simulink subsystem "trial"  (R2023a)
settings: Solver=VariableStepAuto  StartTime=0.0  StopTime=10.0  RelTol=1e-3
undefined symbols (not defined in the file or in its folder): Btrigger_boost, DAapply_nudges, DAdesired_pose, DAff_body_force, DAsolver_weights, Djoy_R_X, Dreverse_throttle, Dthrottle, Iangular_mode, Ilinear_mode
libraries: ros2lib x76
settings Model: Creator=john  LastModifiedBy=john

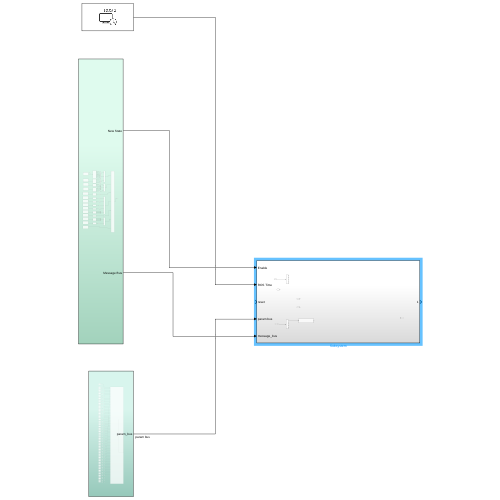
[thumbnail: Simulink's stored preview of the top-level diagram]
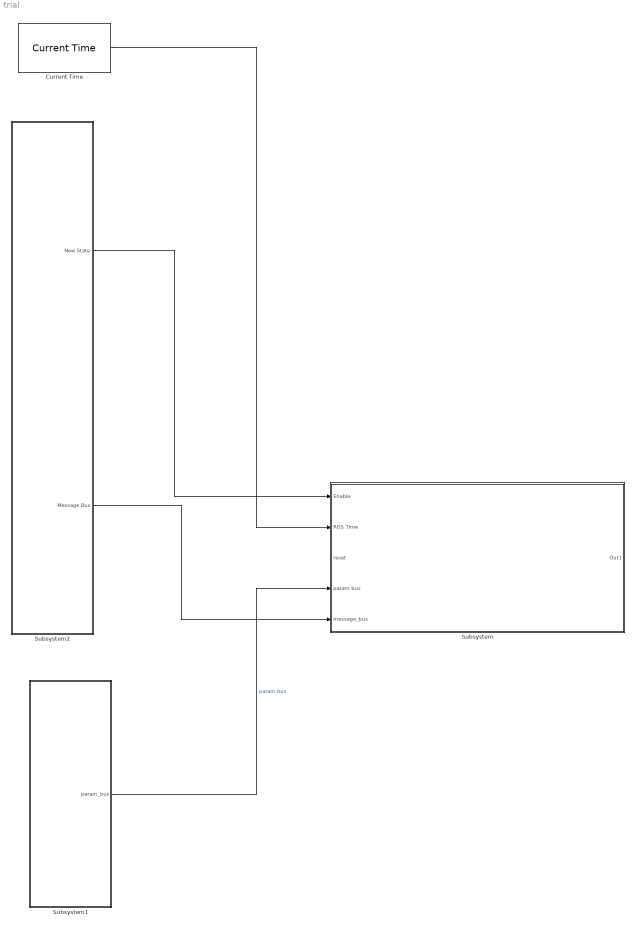
== system trial ==
  Current Time : ros2lib/Current Time  OutputFormat=double  SampleTime=-1  ModelName=complete_controller
  Subsystem : Subsystem
  Subsystem1 : Subsystem
  Subsystem2 : Subsystem
  wires:
  Subsystem2/2(Message Bus) -> Subsystem/5(message_bus)
  Subsystem1/1(param_bus) -> Subsystem/4(param bus)  "param bus"
  Current Time/1 -> Subsystem/2(ROS Time)
  Subsystem2/1(New State) -> Subsystem/1(Enable)

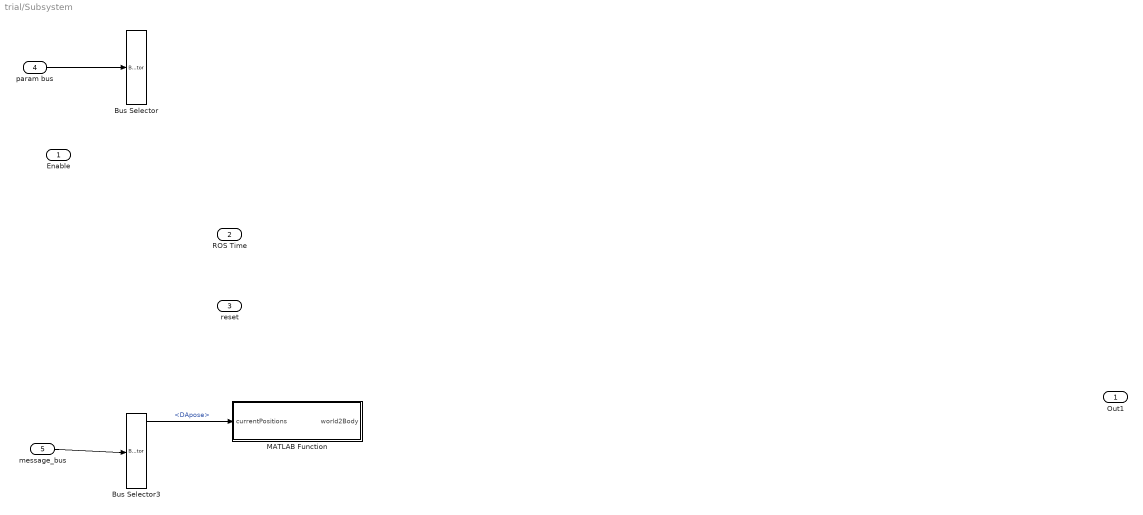
== system trial/Subsystem ==
  Enable : Inport
  ROS Time : Inport  Port=2
  reset : Inport  Port=3
  param bus : Inport  Port=4
  message_bus : Inport  Port=5
  Bus Selector : BusSelector  OutputSignals=DAmax_control,DAp_gains,DAd_gains,DAi_gains,Dreset_threshold
  Bus Selector3 : BusSelector  OutputSignals=current_state.DApose,current_state.DAtwist,desired_pose.DAdesired_pose,Bmotion_enabled
  MATLAB Function : MATLAB Function  TreatAsAtomicUnit=on
  Out1 : Outport
  wires:
  param bus/1 -> Bus Selector/1
  message_bus/1 -> Bus Selector3/1
  Bus Selector3/1 -> MATLAB Function/1(currentPositions)  "<DApose>"

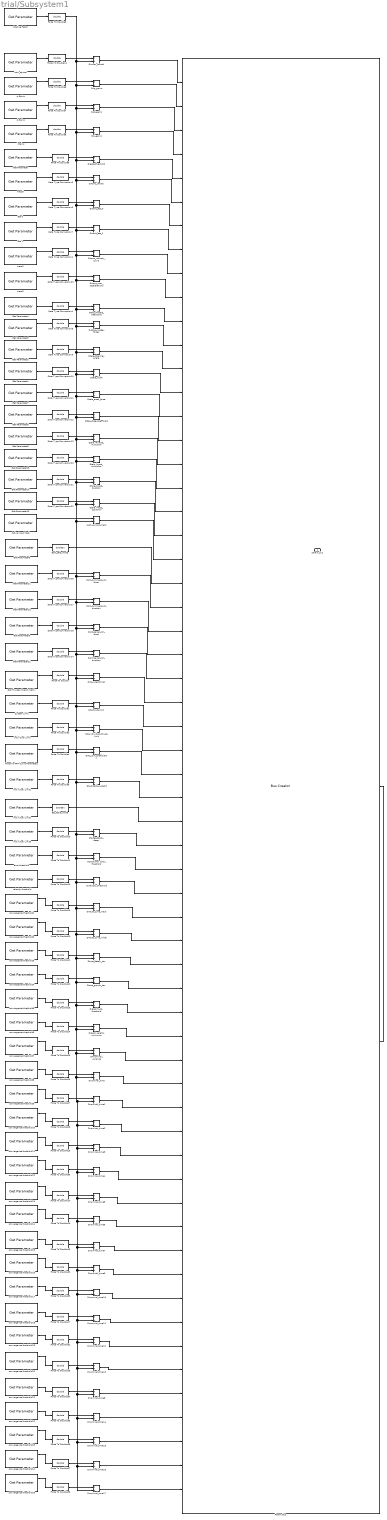
== system trial/Subsystem1 ==
  Active Input Mask : ros2lib/Get Parameter  ParameterName=controller__active_force_mask  ParameterType=int64[]  ParameterMaxArrayLength=6  ParameterInitialValue=[0,0,0,0,0,0]  SampleTime=-1  ModelName=complete_controller  BlockId=ParamGet_complete_controller_223
  Bsnt_safe_mode : DataTypeConversion  OutDataTypeStr=boolean  SaturateOnIntegerOverflow=off  RndMeth=Floor
  Bts_table_mode : DataTypeConversion  OutDataTypeStr=boolean  SaturateOnIntegerOverflow=off  RndMeth=Floor
  DAauto_tune_initial : Product  Inputs=*/
  DAauto_tune_mask : Product  Inputs=*/
  DAd_gains : Product  Inputs=*/
  DAi_gains : Product  Inputs=*/
  DAmax_control : Product  Inputs=*/
  DAnominal_variance : Product  Inputs=*/
  DAp_gains : Product  Inputs=*/
  DAsmc_eta_0 : Product  Inputs=*/
  DAsmc_eta_1 : Product  Inputs=*/
  DAsmc_lamda : Product  Inputs=*/
  DAsmc_max_accelerations : Product  Inputs=*/
  DAsmc_velocity_curve : Product  Inputs=*/
  DAtele_nudge_forces : Product  Inputs=*/
  DAts_rpm_coefficients : Product  Inputs=*/
  DAts_wrenchmat : Product  Inputs=*/
  Data Type Conversion{1,4..14,16..18,20..23} (19 alike) : DataTypeConversion  OutDataTypeStr=double  SaturateOnIntegerOverflow=off  RndMeth=Floor
  Dnominal_time{,1..17} (18 alike) : Product  Inputs=*/
  Dpositional_error_threshold : Product  Inputs=*/
  Dreset_threshold : Product  Inputs=*/
  Dreset_trust_threshold : Product  Inputs=*/
  Dreset_weight_minimum : Product  Inputs=*/
  Dsnt_barrel_roll_duration : Product  Inputs=*/
  Dsnt_barrel_roll_force : Product  Inputs=*/
  Dsnt_summersault_duration : Product  Inputs=*/
  Dsnt_summersault_force : Product  Inputs=*/
  Dtele_accel_force : Product  Inputs=*/
  Dtele_boost_cooldown : Product  Inputs=*/
  Dtele_boost_duration : Product  Inputs=*/
  Dtele_boost_multiplier : Product  Inputs=*/
  Dtele_drag_coefficient : Product  Inputs=*/
  Dtele_reverse_multiplier : Product  Inputs=*/
  Dtele_steering_angle : Product  Inputs=*/
  Dtele_throttle_deadzone : Product  Inputs=*/
  Dtele_width : Product  Inputs=*/
  Dtrust_decay_tau : Product  Inputs=*/
  Dtrust_growth_tau : Product  Inputs=*/
  Dts_disable_weight : Product  Inputs=*/
  Dts_feedback_decay : Product  Inputs=*/
  Dts_individual_thrust_limit : Product  Inputs=*/
  Dts_thrust_limit : Product  Inputs=*/
  Dvelocity_threshold : Product  Inputs=*/
  Eta 0 : ros2lib/Get Parameter  ParameterName=controller__SMC__SMC_params__eta_order_0  ParameterType=int64[]  ParameterMaxArrayLength=6  ParameterInitialValue=0.0  SampleTime=-1  ModelName=complete_controller  BlockId=ParamGet_complete_controller_274
      settings: LibrarySourceBlock=roslib/ROS 2/Get Parameter
  Eta 1 : ros2lib/Get Parameter  ParameterName=controller__SMC__SMC_params__eta_order_1  ParameterType=int64[]  ParameterMaxArrayLength=6  ParameterInitialValue=0.0  SampleTime=-1  ModelName=complete_controller  BlockId=ParamGet_complete_controller_275
      settings: LibrarySourceBlock=roslib/ROS 2/Get Parameter
  Force To Double{,1..38} (39 alike) : DataTypeConversion  OutDataTypeStr=double  SaturateOnIntegerOverflow=off  RndMeth=Floor
  Force To RPM Curve Parameters : ros2lib/Get Parameter  ParameterName=thruster_solver__force_to_rpm_coefficents  ParameterType=int64[]  ParameterMaxArrayLength=8  ParameterInitialValue=[0,0,0,0,0,0,0,0]  SampleTime=-1  ModelName=complete_controller  BlockId=ParamGet_complete_controller_190
      settings: LibrarySourceBlock=roslib/ROS 2/Get Parameter
  Get Parameter : ros2lib/Get Parameter  ParameterName=controller__pid__reset_threshold  ParameterType=int64  ParameterMaxArrayLength=16  ParameterInitialValue=100000  SampleTime=-1  ModelName=complete_controller  BlockId=ParamGet_complete_controller_251
      settings: LibrarySourceBlock=roslib/ROS 2/Get Parameter
  Get Parameter1 : ros2lib/Get Parameter  ParameterName=controller__teleop__width  ParameterType=int64  ParameterMaxArrayLength=16  ParameterInitialValue=900000  SampleTime=-1  ModelName=complete_controller  BlockId=ParamGet_complete_controller_382
  Get Parameter10 : ros2lib/Get Parameter  ParameterName=controller__stunt__summersault_duration  ParameterType=int64  ParameterMaxArrayLength=16  ParameterInitialValue=5000000.0  SampleTime=-1  ModelName=complete_controller  BlockId=ParamGet_complete_controller_425
  Get Parameter11 : ros2lib/Get Parameter  ParameterName=controller__stunt__summersault_force  ParameterType=int64  ParameterMaxArrayLength=16  ParameterInitialValue=20000000  SampleTime=-1  ModelName=complete_controller  BlockId=ParamGet_complete_controller_426
  Get Parameter12 : ros2lib/Get Parameter  ParameterName=controller__stunt__barrel_roll_duration  ParameterType=int64  ParameterMaxArrayLength=16  ParameterInitialValue=4000000.0  SampleTime=-1  ModelName=complete_controller  BlockId=ParamGet_complete_controller_427
  Get Parameter13 : ros2lib/Get Parameter  ParameterName=controller__teleop__boost__cooldown  ParameterType=int64  ParameterMaxArrayLength=16  ParameterInitialValue=10000000  SampleTime=-1  ModelName=complete_controller  BlockId=ParamGet_complete_controller_460
  Get Parameter14 : ros2lib/Get Parameter  ParameterName=controller__teleop__boost__duration  ParameterType=int64  ParameterMaxArrayLength=16  ParameterInitialValue=5000000  SampleTime=-1  ModelName=complete_controller  BlockId=ParamGet_complete_controller_461
  Get Parameter15 : ros2lib/Get Parameter  ParameterName=controller__teleop__boost__multiplier  ParameterType=int64  ParameterMaxArrayLength=16  ParameterInitialValue=1500000  SampleTime=-1  ModelName=complete_controller  BlockId=ParamGet_complete_controller_462
  Get Parameter2 : ros2lib/Get Parameter  ParameterName=controller__teleop__max_steering_angle  ParameterType=int64  ParameterMaxArrayLength=16  ParameterInitialValue=45000000  SampleTime=-1  ModelName=complete_controller  BlockId=ParamGet_complete_controller_383
  Get Parameter3 : ros2lib/Get Parameter  ParameterName=controller__teleop__nudge_forces  ParameterType=int64[]  ParameterMaxArrayLength=6  ParameterInitialValue=[20000000, 20000000, 2000000, 200000, 200000, 2000000]  SampleTime=-1  ModelName=complete_controller  BlockId=ParamGet_complete_controller_384
  Get Parameter4 : ros2lib/Get Parameter  ParameterName=controller__teleop__throttle_deadzone  ParameterType=int64  ParameterMaxArrayLength=16  ParameterInitialValue=50000  SampleTime=-1  ModelName=complete_controller  BlockId=ParamGet_complete_controller_385
  Get Parameter5 : ros2lib/Get Parameter  ParameterName=controller__teleop__reverse_force_multiplier  ParameterType=int64  ParameterMaxArrayLength=16  ParameterInitialValue=400000  SampleTime=-1  ModelName=complete_controller  BlockId=ParamGet_complete_controller_386
  Get Parameter6 : ros2lib/Get Parameter  ParameterName=controller__teleop__drag_coefficient  ParameterType=int64  ParameterMaxArrayLength=16  ParameterInitialValue=420000000  SampleTime=-1  ModelName=complete_controller  BlockId=ParamGet_complete_controller_387
  Get Parameter7 : ros2lib/Get Parameter  ParameterName=controller__teleop__accel_force  ParameterType=int64  ParameterMaxArrayLength=16  ParameterInitialValue=20000000  SampleTime=-1  ModelName=complete_controller  BlockId=ParamGet_complete_controller_388
  Get Parameter8 : ros2lib/Get Parameter  ParameterName=controller__stunt__safe_mode  ParameterType=boolean  ParameterMaxArrayLength=16  ParameterInitialValue=0  SampleTime=-1  ModelName=complete_controller  BlockId=ParamGet_complete_controller_423
  Get Parameter9 : ros2lib/Get Parameter  ParameterName=controller__stunt__barrel_roll_force  ParameterType=int64  ParameterMaxArrayLength=16  ParameterInitialValue=25000000.0  SampleTime=-1  ModelName=complete_controller  BlockId=ParamGet_complete_controller_424
  Get Thruster Wrench Matrix : ros2lib/Get Parameter  ParameterName=talos_wrenchmat  ParameterType=int64[]  ParameterMaxArrayLength=48  ParameterInitialValue=0.0  SampleTime=-1  ModelName=complete_controller  BlockId=ParamGet_complete_controller_191
      settings: LibrarySourceBlock=roslib/ROS 2/Get Parameter
  Iactive_input_mask : Product  Inputs=*/
  Individual Limit : ros2lib/Get Parameter  ParameterName=thruster_solver__individual_thrust_limit  ParameterType=int64  ParameterMaxArrayLength=16  ParameterInitialValue=5.0  SampleTime=-1  ModelName=complete_controller  BlockId=ParamGet_complete_controller_192
      settings: LibrarySourceBlock=roslib/ROS 2/Get Parameter
  Individual Limit1 : ros2lib/Get Parameter  ParameterName=thruster_solver__disable_weight  ParameterType=int64  ParameterMaxArrayLength=16  ParameterInitialValue=10000000  SampleTime=-1  ModelName=complete_controller  BlockId=ParamGet_complete_controller_193
      settings: LibrarySourceBlock=roslib/ROS 2/Get Parameter
  Individual Limit2 : ros2lib/Get Parameter  ParameterName=thruster_solver_table_mode  ParameterType=boolean  ParameterMaxArrayLength=16  ParameterInitialValue=false  SampleTime=-1  ModelName=complete_controller  BlockId=ParamGet_complete_controller_194
      settings: LibrarySourceBlock=roslib/ROS 2/Get Parameter
  Individual Limit3 : ros2lib/Get Parameter  ParameterName=thruster_solver__feedback_decay  ParameterType=int64  ParameterMaxArrayLength=16  ParameterInitialValue=1250000  SampleTime=-1  ModelName=complete_controller  BlockId=ParamGet_complete_controller_486
      settings: LibrarySourceBlock=roslib/ROS 2/Get Parameter
  Param Bus : BusCreator  Inputs=60
  Scaling Factor : ros2lib/Get Parameter  ParameterName=controller__SMC__SMC_params__scaling_factor  ParameterType=int64  ParameterMaxArrayLength=16  ParameterInitialValue=1000000  SampleTime=-1  ModelName=complete_controller  BlockId=ParamGet_complete_controller_219
      settings: LibrarySourceBlock=roslib/ROS 2/Get Parameter
  System Limit : ros2lib/Get Parameter  ParameterName=thruster_solver__system_thrust_limit  ParameterType=int64  ParameterMaxArrayLength=16  ParameterInitialValue=10  SampleTime=-1  ModelName=complete_controller  BlockId=ParamGet_complete_controller_221
      settings: LibrarySourceBlock=roslib/ROS 2/Get Parameter
  convergence threshold1 : ros2lib/Get Parameter  ParameterName=controller__feed_forward__auto_tune__auto_tune_mask  ParameterType=int64[]  ParameterMaxArrayLength=6  ParameterInitialValue=[0;0;0;0;0;0]  SampleTime=-1  ModelName=complete_controller  BlockId=ParamGet_complete_controller_725
      settings: LibrarySourceBlock=roslib/ROS 2/Get Parameter
  convergence threshold10 : ros2lib/Get Parameter  ParameterName=controller__feed_forward__auto_tune__trust_threshold  ParameterType=int64[]  ParameterMaxArrayLength=6  ParameterInitialValue=[970000, 970000, 970000, 970000, 970000, 970000]  SampleTime=-1  ModelName=complete_controller  BlockId=ParamGet_complete_controller_814
      settings: LibrarySourceBlock=roslib/ROS 2/Get Parameter
  convergence threshold11 : ros2lib/Get Parameter  ParameterName=controller__feed_forward__auto_tune__variation_threshold  ParameterType=int64[]  ParameterMaxArrayLength=6  ParameterInitialValue=[1000000, 1000000, 1000000, 1000000, 1000000, 1000000]  SampleTime=-1  ModelName=complete_controller  BlockId=ParamGet_complete_controller_817
      settings: LibrarySourceBlock=roslib/ROS 2/Get Parameter
  convergence threshold12 : ros2lib/Get Parameter  ParameterName=controller__feed_forward__auto_tune__axis_weights  ParameterType=int64[]  ParameterMaxArrayLength=6  ParameterInitialValue=[1000000, 1000000, 1000000, 1000000, 1000000, 1000000]  SampleTime=-1  ModelName=complete_controller  BlockId=ParamGet_complete_controller_820
      settings: LibrarySourceBlock=roslib/ROS 2/Get Parameter
  convergence threshold13 : ros2lib/Get Parameter  ParameterName=controller__feed_forward__auto_tune__variation_der_threshold  ParameterType=int64[]  ParameterMaxArrayLength=6  ParameterInitialValue=[1000000, 1000000, 1000000, 1000000, 1000000, 1000000]  SampleTime=-1  ModelName=complete_controller  BlockId=ParamGet_complete_controller_830
      settings: LibrarySourceBlock=roslib/ROS 2/Get Parameter
  convergence threshold14 : ros2lib/Get Parameter  ParameterName=inertia  ParameterType=int64[]  ParameterMaxArrayLength=3  ParameterInitialValue=[700000,1590000,1650000]  SampleTime=-1  ModelName=complete_controller  BlockId=ParamGet_complete_controller_911
      settings: LibrarySourceBlock=roslib/ROS 2/Get Parameter
  convergence threshold15 : ros2lib/Get Parameter  ParameterName=mass  ParameterType=int64  ParameterMaxArrayLength=6  ParameterInitialValue=32000000  SampleTime=-1  ModelName=complete_controller  BlockId=ParamGet_complete_controller_912
      settings: LibrarySourceBlock=roslib/ROS 2/Get Parameter
  convergence threshold16 : ros2lib/Get Parameter  ParameterName=controller__drag_compensator__apply_mask  ParameterType=int64[]  ParameterMaxArrayLength=36  ParameterInitialValue=zeros(36,1)  SampleTime=-1  ModelName=complete_controller  BlockId=ParamGet_complete_controller_971
      settings: LibrarySourceBlock=roslib/ROS 2/Get Parameter
  convergence threshold17 : ros2lib/Get Parameter  ParameterName=controller__drag_compensator__minimum_samples  ParameterType=int64  ParameterMaxArrayLength=6  ParameterInitialValue=60000000  SampleTime=-1  ModelName=complete_controller  BlockId=ParamGet_complete_controller_972
      settings: LibrarySourceBlock=roslib/ROS 2/Get Parameter
  convergence threshold18 : ros2lib/Get Parameter  ParameterName=controller__drag_compensator__minimum_absolute_velocity  ParameterType=int64  ParameterMaxArrayLength=6  ParameterInitialValue=200000  SampleTime=-1  ModelName=complete_controller  BlockId=ParamGet_complete_controller_973
      settings: LibrarySourceBlock=roslib/ROS 2/Get Parameter
  convergence threshold19 : ros2lib/Get Parameter  ParameterName=controller__drag_compensator__minimum_absolute_positional_error  ParameterType=int64  ParameterMaxArrayLength=3  ParameterInitialValue=200000  SampleTime=-1  ModelName=complete_controller  BlockId=ParamGet_complete_controller_974
      settings: LibrarySourceBlock=roslib/ROS 2/Get Parameter
  convergence threshold2 : ros2lib/Get Parameter  ParameterName=auto_ff__auto_ff  ParameterType=int64[]  ParameterMaxArrayLength=6  ParameterInitialValue=[0;0;0;0;0;0]  SampleTime=-1  ModelName=complete_controller  BlockId=ParamGet_complete_controller_730
      settings: LibrarySourceBlock=roslib/ROS 2/Get Parameter
  convergence threshold20 : ros2lib/Get Parameter  ParameterName=controller__drag_compensator__minimum_average_sampled_velocity  ParameterType=int64[]  ParameterMaxArrayLength=6  ParameterInitialValue=[100000,100000,100000,100000,100000,100000]  SampleTime=-1  ModelName=complete_controller  BlockId=ParamGet_complete_controller_975
      settings: LibrarySourceBlock=roslib/ROS 2/Get Parameter
  convergence threshold21 : ros2lib/Get Parameter  ParameterName=controller__drag_compensator__minimum_R2_coeffiecent  ParameterType=int64  ParameterMaxArrayLength=6  ParameterInitialValue=700000  SampleTime=-1  ModelName=complete_controller  BlockId=ParamGet_complete_controller_978
      settings: LibrarySourceBlock=roslib/ROS 2/Get Parameter
  convergence threshold22 : ros2lib/Get Parameter  ParameterName=controller__drag_compensator__learning_rate  ParameterType=int64  ParameterMaxArrayLength=6  ParameterInitialValue=200000  SampleTime=-1  ModelName=complete_controller  BlockId=ParamGet_complete_controller_981
      settings: LibrarySourceBlock=roslib/ROS 2/Get Parameter
  convergence threshold23 : ros2lib/Get Parameter  ParameterName=controller__drag_compensator__initial_compensation__forward  ParameterType=int64[]  ParameterMaxArrayLength=36  ParameterInitialValue=zeros(36,1)  SampleTime=-1  ModelName=complete_controller  BlockId=ParamGet_complete_controller_1006
      settings: LibrarySourceBlock=roslib/ROS 2/Get Parameter
  convergence threshold24 : ros2lib/Get Parameter  ParameterName=controller__autoff__initial_ff  ParameterType=int64[]  ParameterMaxArrayLength=6  ParameterInitialValue=[0,0,0,0,0,0,0]  SampleTime=-1  ModelName=complete_controller  BlockId=ParamGet_complete_controller_1009
      settings: LibrarySourceBlock=roslib/ROS 2/Get Parameter
  convergence threshold25 : ros2lib/Get Parameter  ParameterName=controller__drag_compensator__initial_compensation__reverse  ParameterType=int64[]  ParameterMaxArrayLength=36  ParameterInitialValue=zeros(36,1)  SampleTime=-1  ModelName=complete_controller  BlockId=ParamGet_complete_controller_1030
      settings: LibrarySourceBlock=roslib/ROS 2/Get Parameter
  convergence threshold3 : ros2lib/Get Parameter  ParameterName=controller__controller_scale__trust_decay_tau  ParameterType=int64  ParameterMaxArrayLength=6  ParameterInitialValue=1000000  SampleTime=-1  ModelName=complete_controller  BlockId=ParamGet_complete_controller_760
      settings: LibrarySourceBlock=roslib/ROS 2/Get Parameter
  convergence threshold4 : ros2lib/Get Parameter  ParameterName=controller__controller_scale__trust_growth_tau  ParameterType=int64  ParameterMaxArrayLength=6  ParameterInitialValue=1000000  SampleTime=-1  ModelName=complete_controller  BlockId=ParamGet_complete_controller_763
      settings: LibrarySourceBlock=roslib/ROS 2/Get Parameter
  convergence threshold5 : ros2lib/Get Parameter  ParameterName=controller__controller_scale__reset_trust_threshold  ParameterType=int64  ParameterMaxArrayLength=200000  ParameterInitialValue=200000  SampleTime=-1  ModelName=complete_controller  BlockId=ParamGet_complete_controller_766
      settings: LibrarySourceBlock=roslib/ROS 2/Get Parameter
  convergence threshold6 : ros2lib/Get Parameter  ParameterName=controller__controller_scale__reset_weight_minimum  ParameterType=int64  ParameterMaxArrayLength=6  ParameterInitialValue=3000000  SampleTime=-1  ModelName=complete_controller  BlockId=ParamGet_complete_controller_769
      settings: LibrarySourceBlock=roslib/ROS 2/Get Parameter
  convergence threshold7 : ros2lib/Get Parameter  ParameterName=controller__controller_scale__nominal_variance  ParameterType=int64[]  ParameterMaxArrayLength=6  ParameterInitialValue=[0;0;0;0;0;0]  SampleTime=-1  ModelName=complete_controller  BlockId=ParamGet_complete_controller_772
      settings: LibrarySourceBlock=roslib/ROS 2/Get Parameter
  convergence threshold8 : ros2lib/Get Parameter  ParameterName=controller__controller_scale__nominal_time  ParameterType=int64  ParameterMaxArrayLength=6  ParameterInitialValue=3000000  SampleTime=-1  ModelName=complete_controller  BlockId=ParamGet_complete_controller_775
      settings: LibrarySourceBlock=roslib/ROS 2/Get Parameter
  convergence threshold9 : ros2lib/Get Parameter  ParameterName=controller__feed_forward__auto_tune__decay_factor  ParameterType=int64[]  ParameterMaxArrayLength=6  ParameterInitialValue=[200000, 200000, 200000, 200000, 200000, 200000]  SampleTime=-1  ModelName=complete_controller  BlockId=ParamGet_complete_controller_805
      settings: LibrarySourceBlock=roslib/ROS 2/Get Parameter
  d Gains : ros2lib/Get Parameter  ParameterName=controller__PID__d_gains  ParameterType=int64[]  ParameterMaxArrayLength=6  ParameterInitialValue=[0,0,0,0,0,0]  SampleTime=-1  ModelName=complete_controller  BlockId=ParamGet_complete_controller_260
      settings: LibrarySourceBlock=roslib/ROS 2/Get Parameter
  error threshold : ros2lib/Get Parameter  ParameterName=controller__feed_forward__auto_tune__positional_error_threshold  ParameterType=int64  ParameterMaxArrayLength=16  ParameterInitialValue=100000  SampleTime=-1  ModelName=complete_controller  BlockId=ParamGet_complete_controller_702
      settings: LibrarySourceBlock=roslib/ROS 2/Get Parameter
  i Gains : ros2lib/Get Parameter  ParameterName=controller__PID__i_gains  ParameterType=int64[]  ParameterMaxArrayLength=6  ParameterInitialValue=[0,0,0,0,0,0]  SampleTime=-1  ModelName=complete_controller  BlockId=ParamGet_complete_controller_261
      settings: LibrarySourceBlock=roslib/ROS 2/Get Parameter
  mass1 : ros2lib/Get Parameter  ParameterName=controller__SMC__SMC_params__velocity_curve_params  ParameterType=int64[]  ParameterMaxArrayLength=12  ParameterInitialValue=[0,0,0,0,0,0,0,0,0,0,0,0]  SampleTime=-1  ModelName=complete_controller  BlockId=ParamGet_complete_controller_276
      settings: LibrarySourceBlock=roslib/ROS 2/Get Parameter
  mass2 : ros2lib/Get Parameter  ParameterName=controller__SMC__max_target_accelerations  ParameterType=int64[]  ParameterMaxArrayLength=6  ParameterInitialValue=[10000,10000,10000,10000,10000,10000]  SampleTime=-1  ModelName=complete_controller  BlockId=ParamGet_complete_controller_467
      settings: LibrarySourceBlock=roslib/ROS 2/Get Parameter
  mass5 : ros2lib/Get Parameter  ParameterName=controller__SMC__SMC_params__lambda  ParameterType=int64[]  ParameterMaxArrayLength=6  ParameterInitialValue=0.0  SampleTime=-1  ModelName=complete_controller  BlockId=ParamGet_complete_controller_278
      settings: LibrarySourceBlock=roslib/ROS 2/Get Parameter
  max_control : ros2lib/Get Parameter  ParameterName=controller__PID__max_control_thresholds  ParameterType=int64[]  ParameterMaxArrayLength=6  ParameterInitialValue=[0,0,0,0,0,0]  SampleTime=-1  ModelName=complete_controller  BlockId=ParamGet_complete_controller_262
      settings: LibrarySourceBlock=roslib/ROS 2/Get Parameter
  p Gains : ros2lib/Get Parameter  ParameterName=controller__PID__p_gains  ParameterType=int64[]  ParameterMaxArrayLength=6  ParameterInitialValue=[0,0,0,0,0,0]  SampleTime=-1  ModelName=complete_controller  BlockId=ParamGet_complete_controller_263
      settings: LibrarySourceBlock=roslib/ROS 2/Get Parameter
  velocity threshold : ros2lib/Get Parameter  ParameterName=controller__feed_forward__auto_tune__velocity_threshold  ParameterType=int64  ParameterMaxArrayLength=16  ParameterInitialValue=100000  SampleTime=-1  ModelName=complete_controller  BlockId=ParamGet_complete_controller_703
      settings: LibrarySourceBlock=roslib/ROS 2/Get Parameter
  param_bus : Outport
  wires:
  Data Type Conversion10/1 -> Dtele_width/1
  Get Parameter4/1 -> Data Type Conversion4/1
  Data Type Conversion22/1 -> Dtele_boost_cooldown/1
  Data Type Conversion20/1 -> Dtele_boost_multiplier/1
  Data Type Conversion11/1 -> Dtele_accel_force/1
  Data Type Conversion23/1 -> DAsmc_max_accelerations/1
  Get Parameter11/1 -> Data Type Conversion16/1
  Get Parameter5/1 -> Data Type Conversion13/1
  Force To RPM Curve Parameters/1 -> Force To Double4/1
  Data Type Conversion13/1 -> Dtele_reverse_multiplier/1
  Get Parameter7/1 -> Data Type Conversion11/1
  Get Parameter1/1 -> Data Type Conversion10/1
  Data Type Conversion21/1 -> Dtele_boost_duration/1
  Get Parameter12/1 -> Data Type Conversion14/1
  Data Type Conversion16/1 -> Dsnt_summersault_force/1
  Scaling Factor/1 -> Force To Double3/1
  Get Parameter6/1 -> Data Type Conversion12/1
  Eta 0/1 -> Data Type Conversion6/1
  Data Type Conversion7/1 -> DAsmc_eta_1/1
  Individual Limit/1 -> Force To Double2/1
  Data Type Conversion8/1 -> DAtele_nudge_forces/1
  Force To Double6/1 -> DAp_gains/1
  p Gains/1 -> Force To Double6/1
  Force To Double5/1 -> Dts_disable_weight/1
  Get Thruster Wrench Matrix/1 -> Force To Double/1
  Get Parameter10/1 -> Data Type Conversion17/1
  Data Type Conversion18/1 -> Dsnt_barrel_roll_force/1
  max_control/1 -> Force To Double11/1
  mass2/1 -> Data Type Conversion23/1
  Get Parameter13/1 -> Data Type Conversion22/1
  Data Type Conversion14/1 -> Dsnt_barrel_roll_duration/1
  Force To Double8/1 -> DAi_gains/1
  Active Input Mask/1 -> Iactive_input_mask/1
  Eta 1/1 -> Data Type Conversion7/1
  Force To Double7/1 -> DAd_gains/1
  Data Type Conversion12/1 -> Dtele_drag_coefficient/1
  d Gains/1 -> Force To Double7/1
  Force To Double4/1 -> DAts_rpm_coefficients/1
  Get Parameter9/1 -> Data Type Conversion18/1
  Get Parameter8/1 -> Bsnt_safe_mode/1
  Individual Limit1/1 -> Force To Double5/1
  Data Type Conversion5/1 -> DAsmc_lamda/1
  mass1/1 -> Data Type Conversion1/1
  Get Parameter/1 -> Force To Double9/1
  Data Type Conversion9/1 -> Dtele_steering_angle/1
  Individual Limit3/1 -> Force To Double10/1
  Get Parameter14/1 -> Data Type Conversion21/1
  mass5/1 -> Data Type Conversion5/1
  System Limit/1 -> Force To Double1/1
  Get Parameter3/1 -> Data Type Conversion8/1
  i Gains/1 -> Force To Double8/1
  Force To Double11/1 -> DAmax_control/1
  Data Type Conversion1/1 -> DAsmc_velocity_curve/1
  Get Parameter15/1 -> Data Type Conversion20/1
  Force To Double1/1 -> Dts_thrust_limit/1
  Data Type Conversion4/1 -> Dtele_throttle_deadzone/1
  Get Parameter2/1 -> Data Type Conversion9/1
  Force To Double9/1 -> Dreset_threshold/1
  Force To Double2/1 -> Dts_individual_thrust_limit/1
  Force To Double10/1 -> Dts_feedback_decay/1
  Data Type Conversion17/1 -> Dsnt_summersault_duration/1
  Data Type Conversion6/1 -> DAsmc_eta_0/1
  Force To Double/1 -> DAts_wrenchmat/1
  Individual Limit2/1 -> Bts_table_mode/1
  Dts_feedback_decay/1 -> Param Bus/33  "Dts_feedback_decay"
  Bts_table_mode/1 -> Param Bus/32  "Bts_table_mode"
  Dts_disable_weight/1 -> Param Bus/31  "Dts_disable_weight"
  DAts_rpm_coefficients/1 -> Param Bus/30  "DAts_rpm_coefficients"
  Dts_individual_thrust_limit/1 -> Param Bus/29  "Dts_individual_thrust_limit"
  Dts_thrust_limit/1 -> Param Bus/28  "Dts_thrust_limit"
  DAts_wrenchmat/1 -> Param Bus/27  "DAts_wrenchmat"
  Dsnt_barrel_roll_duration/1 -> Param Bus/26  "Dsnt_barrel_roll_duration"
  Bsnt_safe_mode/1 -> Param Bus/22  "Bsnt_safe_mode"
  Dsnt_barrel_roll_force/1 -> Param Bus/25  "Dsnt_barrel_roll_force"
  Dsnt_summersault_duration/1 -> Param Bus/24  "Dsnt_summersault_duration"
  Dsnt_summersault_force/1 -> Param Bus/23  "Dsnt_summersault_force"
  Iactive_input_mask/1 -> Param Bus/21  "Iactive_input_mask"
  Dtele_boost_cooldown/1 -> Param Bus/20  "Dtele_boost_cooldown"
  Dtele_boost_duration/1 -> Param Bus/19  "Dtele_boost_duration"
  Dtele_boost_multiplier/1 -> Param Bus/18  "Dtele_boost_multiplier"
  Dtele_reverse_multiplier/1 -> Param Bus/17  "Dtele_reverse_multiplier"
  Dtele_drag_coefficient/1 -> Param Bus/16  "Dtele_drag_coefficient"
  Dtele_accel_force/1 -> Param Bus/15  "Dtele_accel_force"
  Dtele_width/1 -> Param Bus/14  "Dtele_width"
  Dtele_steering_angle/1 -> Param Bus/13  "Dtele_steering_angle"
  DAtele_nudge_forces/1 -> Param Bus/12  "DAtele_nudge_forces"
  Dtele_throttle_deadzone/1 -> Param Bus/11  "Dtele_throttle_deadzone"
  DAsmc_max_accelerations/1 -> Param Bus/10  "DAsmc_max_accelerations"
  DAsmc_velocity_curve/1 -> Param Bus/9  "DAsmc_velocity_curve"
  DAsmc_eta_1/1 -> Param Bus/8  "DAsmc_eta_1"
  DAsmc_eta_0/1 -> Param Bus/7  "DAsmc_eta_0"
  DAsmc_lamda/1 -> Param Bus/6  "DAsmc_lamda"
  Dreset_threshold/1 -> Param Bus/5  "Dreset_threshold"
  DAi_gains/1 -> Param Bus/4  "DAi_gains"
  DAd_gains/1 -> Param Bus/3  "DAd_gains"
  DAp_gains/1 -> Param Bus/2  "DAp_gains"
  DAmax_control/1 -> Param Bus/1  "DAmax_control"
  Param Bus/1 -> param_bus/1
  error threshold/1 -> Force To Double12/1
  velocity threshold/1 -> Force To Double13/1
  Dpositional_error_threshold/1 -> Param Bus/34  "Dpositional_error_threshold"
  Dvelocity_threshold/1 -> Param Bus/35  "Dvelocity_threshold"
  convergence threshold1/1 -> Force To Double19/1
  DAauto_tune_mask/1 -> Param Bus/36  "DAauto_tune_mask"
  Force To Double13/1 -> Dvelocity_threshold/1
  Force To Double12/1 -> Dpositional_error_threshold/1
  Force To Double19/1 -> DAauto_tune_mask/1
  convergence threshold2/1 -> Force To Double20/1
  DAauto_tune_initial/1 -> Param Bus/37  "DAauto_tune_initial"
  Force To Double20/1 -> DAauto_tune_initial/1
  convergence threshold3/1 -> Force To Double21/1
  Dtrust_decay_tau/1 -> Param Bus/38  "Dtrust_decay_tau"
  Force To Double21/1 -> Dtrust_decay_tau/1
  convergence threshold4/1 -> Force To Double22/1
  Dtrust_growth_tau/1 -> Param Bus/39  "Dtrust_growth_tau"
  Force To Double22/1 -> Dtrust_growth_tau/1
  convergence threshold5/1 -> Force To Double23/1
  Dreset_trust_threshold/1 -> Param Bus/40  "Dreset_trust_threshold"
  Force To Double23/1 -> Dreset_trust_threshold/1
  convergence threshold6/1 -> Force To Double24/1
  Dreset_weight_minimum/1 -> Param Bus/41  "Dreset_weight_minimum"
  Force To Double24/1 -> Dreset_weight_minimum/1
  convergence threshold7/1 -> Force To Double25/1
  DAnominal_variance/1 -> Param Bus/42  "DAnominal_variance"
  Force To Double25/1 -> DAnominal_variance/1
  convergence threshold8/1 -> Force To Double26/1
  Dnominal_time/1 -> Param Bus/43  "Dnominal_time"
  Force To Double26/1 -> Dnominal_time/1
  convergence threshold9/1 -> Force To Double27/1
  Force To Double27/1 -> Dnominal_time1/1
  convergence threshold10/1 -> Force To Double28/1
  Force To Double28/1 -> Dnominal_time2/1
  convergence threshold11/1 -> Force To Double29/1
  Force To Double29/1 -> Dnominal_time3/1
  convergence threshold12/1 -> Force To Double30/1
  Force To Double30/1 -> Dnominal_time4/1
  Dnominal_time1/1 -> Param Bus/44  "DAautoff_body_force_decay_percentage"
  Dnominal_time2/1 -> Param Bus/45  "DAautoff_measurement_trust_threshold"
  Dnominal_time3/1 -> Param Bus/46  "DAautoff_standard_variation_threshold"
  Dnominal_time4/1 -> Param Bus/47  "DAautoff_active_force_weights"
  convergence threshold13/1 -> Force To Double14/1
  Force To Double14/1 -> Dnominal_time5/1
  Dnominal_time5/1 -> Param Bus/48  "DAautoff_variation_derivative_threshold"
  Force To Double16/1 -> Dnominal_time6/1
  Dnominal_time6/1 -> Param Bus/49  "DAinterias"
  convergence threshold15/1 -> Force To Double15/1
  Dnominal_time7/1 -> Param Bus/50  "Dmass"
  Force To Double15/1 -> Dnominal_time7/1
  convergence threshold14/1 -> Force To Double16/1
  Dnominal_time13/1 -> Param Bus/55  "DAminimum_drag_update_velocity"
  convergence threshold20/1 -> Force To Double18/1
  Dnominal_time10/1 -> Param Bus/52  "Iminimum_drag_samples"
  Force To Double31/1 -> Dnominal_time12/1
  Dnominal_time11/1 -> Param Bus/53  "Dminimum_drag_sampling_velocity"
  convergence threshold19/1 -> Force To Double31/1
  convergence threshold18/1 -> Force To Double17/1
  Force To Double33/1 -> Dnominal_time10/1
  Dnominal_time12/1 -> Param Bus/54  "Dminimum_drag_positional_error"
  Dnominal_time9/1 -> Param Bus/51  "IAdrag_apply_mask"
  Force To Double17/1 -> Dnominal_time11/1
  convergence threshold17/1 -> Force To Double33/1
  Force To Double32/1 -> Dnominal_time9/1
  convergence threshold16/1 -> Force To Double32/1
  Force To Double18/1 -> Dnominal_time13/1
  convergence threshold21/1 -> Force To Double34/1
  Force To Double34/1 -> Dnominal_time8/1
  Dnominal_time8/1 -> Param Bus/56  "Ddrag_minimum_correspondence_coeffiecent"
  convergence threshold22/1 -> Force To Double35/1
  Dnominal_time14/1 -> Param Bus/57  "Ddrag_learning_rate"
  Force To Double35/1 -> Dnominal_time14/1
  convergence threshold23/1 -> Force To Double36/1
  Dnominal_time15/1 -> Param Bus/58  "DAdrag_init_compensation_forward"
  Force To Double36/1 -> Dnominal_time15/1
  Dnominal_time16/1 -> Param Bus/59  "DAautoff_init_compensation"
  Force To Double37/1 -> Dnominal_time16/1
  convergence threshold24/1 -> Force To Double37/1
  Force To Double3/1 -> Dtele_throttle_deadzone/2, DAtele_nudge_forces/2, Dtele_steering_angle/2, Dtele_width/2, Dtele_accel_force/2, Dtele_drag_coefficient/2, Dtele_boost_multiplier/2, Dtele_boost_duration/2, Dtele_boost_cooldown/2, Dsnt_summersault_force/2, Dsnt_summersault_duration/2, Dsnt_barrel_roll_duration/2, DAts_wrenchmat/2, Dts_thrust_limit/2, Dts_individual_thrust_limit/2, DAts_rpm_coefficients/2, Dvelocity_threshold/2, Dtrust_decay_tau/2, Dtrust_growth_tau/2, Dreset_trust_threshold/2, Dreset_weight_minimum/2, DAnominal_variance/2, Dnominal_time17/2, Dnominal_time16/2, Dnominal_time15/2, Dnominal_time14/2, Dnominal_time8/2, Dnominal_time13/2, Dnominal_time12/2, Dnominal_time11/2, Dnominal_time10/2, Dnominal_time9/2, Dnominal_time7/2, Dnominal_time6/2, Dnominal_time5/2, Dnominal_time4/2, Dnominal_time3/2, Dnominal_time2/2, Dnominal_time1/2, Dnominal_time/2, DAauto_tune_initial/2, DAauto_tune_mask/2, Dpositional_error_threshold/2, Dts_feedback_decay/2, Dts_disable_weight/2, Dsnt_barrel_roll_force/2, Iactive_input_mask/2, Dtele_reverse_multiplier/2, DAsmc_max_accelerations/2, DAsmc_velocity_curve/2, DAsmc_eta_1/2, DAsmc_eta_0/2, DAsmc_lamda/2, Dreset_threshold/2, DAi_gains/2, DAd_gains/2, DAp_gains/2, DAmax_control/2
  Force To Double38/1 -> Dnominal_time17/1
  convergence threshold25/1 -> Force To Double38/1
  Dnominal_time17/1 -> Param Bus/60  "DAdrag_init_compensation_reverse"

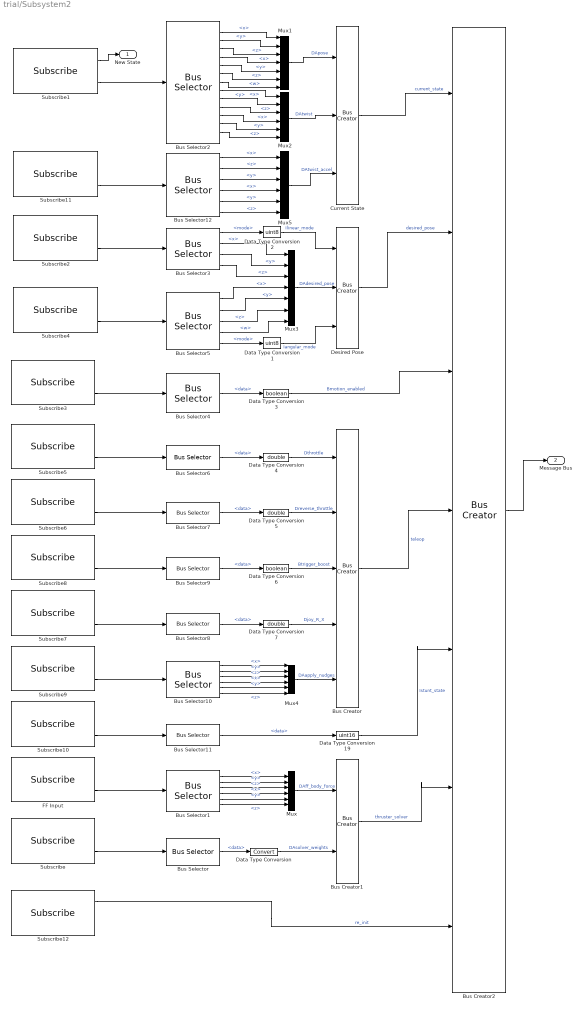
== system trial/Subsystem2 ==
  Bus Creator : BusCreator  Inputs=Dthrottle,Dreverse_throttle,Btrigger_boost,Djoy_R_X,DAapply_nudges
  Bus Creator1 : BusCreator  Inputs=DAff_body_force,DAsolver_weights
  Bus Creator2 : BusCreator  Inputs=7
  Bus Selector{,4,6..9,11} (7 alike) : BusSelector  OutputSignals=data
  Bus Selector1 : BusSelector  OutputSignals=linear.x,linear.y,linear.z,angular.x,angular.y,angular.z
  Bus Selector10 : BusSelector  OutputSignals=linear.x,linear.y,linear.z,angular.x,angular.y,angular.z
  Bus Selector12 : BusSelector  OutputSignals=accel.accel.linear.x,accel.accel.linear.z,accel.accel.linear.y,accel.accel.angular.x,accel.accel.angular.y,accel.accel.angular.z
  Bus Selector2 : BusSelector  OutputSignals=pose.pose.position.x,pose.pose.position.y,pose.pose.position.z,pose.pose.orientation.x,pose.pose.orientation.y,pose.pose.orientation.z,pose.pose.orientation.w,twist.twist.linear.x,twist.twist.linear.y,twist.twist.linear.z,twist.twist.angular.x,twist.twist.angular.y,twist.twist.angular.z
  Bus Selector3 : BusSelector  OutputSignals=mode,setpoint_vect.x,setpoint_vect.y,setpoint_vect.z
  Bus Selector5 : BusSelector  OutputSignals=setpoint_quat.x,setpoint_quat.y,setpoint_quat.z,setpoint_quat.w,mode
  Current State : BusCreator  Inputs=3
  Data Type Conversion : DataTypeConversion  SaturateOnIntegerOverflow=off  RndMeth=Floor
  Data Type Conversion1 : DataTypeConversion  OutDataTypeStr=uint8  SaturateOnIntegerOverflow=off  RndMeth=Floor
  Data Type Conversion19 : DataTypeConversion  OutDataTypeStr=uint16  SaturateOnIntegerOverflow=off  RndMeth=Floor
  Data Type Conversion2 : DataTypeConversion  OutDataTypeStr=uint8  SaturateOnIntegerOverflow=off  RndMeth=Floor
  Data Type Conversion3 : DataTypeConversion  OutDataTypeStr=boolean  SaturateOnIntegerOverflow=off  RndMeth=Floor
  Data Type Conversion4 : DataTypeConversion  OutDataTypeStr=double  SaturateOnIntegerOverflow=off  RndMeth=Floor
  Data Type Conversion5 : DataTypeConversion  OutDataTypeStr=double  SaturateOnIntegerOverflow=off  RndMeth=Floor
  Data Type Conversion6 : DataTypeConversion  OutDataTypeStr=boolean  SaturateOnIntegerOverflow=off  RndMeth=Floor
  Data Type Conversion7 : DataTypeConversion  OutDataTypeStr=double  SaturateOnIntegerOverflow=off  RndMeth=Floor
  Desired Pose : BusCreator  Inputs=Ilinear_mode,DAdesired_pose,Iangular_mode
  FF Input : ros2lib/Subscribe  topicSource=Specify your own  topic=/talos/controller/FF_body_force  messageType=geometry_msgs/Twist  sampleTime=-1  QOSHistory=Keep last  QOSDepth=1  QOSReliability=Reliable  QOSDurability=Volatile
      settings: LibrarySourceBlock=roslib/ROS 2/Subscribe
  Mux{,2,4..5} (4 alike) : Mux  Inputs=6
  Mux1 : Mux  Inputs=7
  Mux3 : Mux  Inputs=7
  Subscribe : ros2lib/Subscribe  topicSource=Specify your own  topic=/talos/controller/solver_weights  messageType=std_msgs/Int32MultiArray  sampleTime=-1  QOSHistory=Keep last  QOSDepth=1  QOSReliability=Reliable  QOSDurability=Volatile
      settings: LibrarySourceBlock=roslib/ROS 2/Subscribe
  Subscribe1 : ros2lib/Subscribe  topicSource=Specify your own  topic=/talos/odometry/filtered  messageType=nav_msgs/Odometry  sampleTime=-1  QOSHistory=Keep last  QOSDepth=1  QOSReliability=Reliable  QOSDurability=Volatile
      settings: LibrarySourceBlock=roslib/ROS 2/Subscribe
  Subscribe10 : ros2lib/Subscribe  topicSource=Specify your own  topic=/talos/controller/stunt_state  messageType=std_msgs/UInt16  sampleTime=-1  QOSHistory=Keep last  QOSDepth=1  QOSReliability=Reliable  QOSDurability=Volatile
  Subscribe11 : ros2lib/Subscribe  topicSource=Specify your own  topic=/talos/accel/filtered  messageType=geometry_msgs/AccelWithCovarianceStamped  sampleTime=-1  QOSHistory=Keep last  QOSDepth=1  QOSReliability=Reliable  QOSDurability=Volatile
      settings: LibrarySourceBlock=roslib/ROS 2/Subscribe
  Subscribe12 : ros2lib/Subscribe  topicSource=Specify your own  topic=/talos/controller/re_init_accumulators  messageType=std_msgs/Empty  sampleTime=-1  QOSHistory=Keep last  QOSDepth=1  QOSReliability=Reliable  QOSDurability=Volatile
      settings: LibrarySourceBlock=roslib/ROS 2/Subscribe
  Subscribe2 : ros2lib/Subscribe  topicSource=Specify your own  topic=/talos/controller/linear  messageType=riptide_msgs2/ControllerCommand  sampleTime=-1  QOSHistory=Keep last  QOSDepth=1  QOSReliability=Reliable  QOSDurability=Volatile
      settings: LibrarySourceBlock=roslib/ROS 2/Subscribe
  Subscribe3 : ros2lib/Subscribe  topicSource=Specify your own  topic=/talos/controller/motion_enabled  messageType=std_msgs/Bool  sampleTime=-1  QOSHistory=Keep last  QOSDepth=1  QOSReliability=Reliable  QOSDurability=Volatile
      settings: LibrarySourceBlock=roslib/ROS 2/Subscribe
  Subscribe4 : ros2lib/Subscribe  topicSource=Specify your own  topic=/talos/controller/angular  messageType=riptide_msgs2/ControllerCommand  sampleTime=-1  QOSHistory=Keep last  QOSDepth=1  QOSReliability=Reliable  QOSDurability=Volatile
      settings: LibrarySourceBlock=roslib/ROS 2/Subscribe
  Subscribe5 : ros2lib/Subscribe  topicSource=Specify your own  topic=/talos/teleop/throttle  messageType=std_msgs/Float32  sampleTime=-1  QOSHistory=Keep last  QOSDepth=5  QOSReliability=Best effort  QOSDurability=Volatile
  Subscribe6 : ros2lib/Subscribe  topicSource=Specify your own  topic=/talos/teleop/reverse  messageType=std_msgs/Float32  sampleTime=-1  QOSHistory=Keep last  QOSDepth=5  QOSReliability=Best effort  QOSDurability=Volatile
  Subscribe7 : ros2lib/Subscribe  topicSource=Specify your own  topic=/talos/teleop/joy_R_X  messageType=std_msgs/Float32  sampleTime=-1  QOSHistory=Keep last  QOSDepth=5  QOSReliability=Best effort  QOSDurability=Volatile
  Subscribe8 : ros2lib/Subscribe  topicSource=Specify your own  topic=/talos/teleop/trigger_boost  messageType=std_msgs/Bool  sampleTime=-1  QOSHistory=Keep last  QOSDepth=1  QOSReliability=Reliable  QOSDurability=Volatile
  Subscribe9 : ros2lib/Subscribe  topicSource=Specify your own  topic=/talos/teleop/apply_nudges  messageType=geometry_msgs/Twist  sampleTime=-1  QOSHistory=Keep last  QOSDepth=5  QOSReliability=Best effort  QOSDurability=Volatile
  New State : Outport
  Message Bus : Outport  Port=2
  wires:
  Bus Selector1/1 -> Mux/1  "<x>"
  Bus Selector2/4 -> Mux1/4  "<x>"
  Mux/1 -> Bus Creator1/1  "DAff_body_force"
  Bus Selector2/12 -> Mux2/5  "<y>"
  Bus Selector11/1 -> Data Type Conversion19/1  "<data>"
  Subscribe4/2 -> Bus Selector5/1
  Bus Selector2/1 -> Mux1/1  "<x>"
  Bus Selector2/5 -> Mux1/5  "<y>"
  Bus Selector5/4 -> Mux3/7  "<w>"
  Subscribe10/2 -> Bus Selector11/1
  Bus Selector/1 -> Data Type Conversion/1  "<data>"
  Bus Selector2/7 -> Mux1/7  "<w>"
  Bus Selector10/6 -> Mux4/6  "<z>"
  Subscribe9/2 -> Bus Selector10/1
  Bus Selector2/9 -> Mux2/2  "<y>"
  Bus Selector1/4 -> Mux/4  "<x>"
  Bus Selector10/5 -> Mux4/5  "<y>"
  Subscribe3/2 -> Bus Selector4/1
  Bus Selector5/2 -> Mux3/5  "<y>"
  Bus Selector10/4 -> Mux4/4  "<x>"
  Bus Selector5/1 -> Mux3/4  "<x>"
  Bus Selector2/11 -> Mux2/4  "<x>"
  Subscribe7/2 -> Bus Selector8/1
  Bus Selector3/3 -> Mux3/2  "<y>"
  Bus Selector8/1 -> Data Type Conversion7/1  "<data>"
  Bus Selector3/4 -> Mux3/3  "<z>"
  Bus Selector5/3 -> Mux3/6  "<z>"
  Bus Selector7/1 -> Data Type Conversion5/1  "<data>"
  Subscribe1/1 -> New State/1
  Mux4/1 -> Bus Creator/5  "DAapply_nudges"
  Subscribe6/2 -> Bus Selector7/1
  Bus Selector3/2 -> Mux3/1  "<x>"
  Bus Selector10/3 -> Mux4/3  "<z>"
  Bus Selector2/13 -> Mux2/6  "<z>"
  Subscribe2/2 -> Bus Selector3/1
  Subscribe1/2 -> Bus Selector2/1
  Bus Selector1/2 -> Mux/2  "<y>"
  Data Type Conversion/1 -> Bus Creator1/2  "DAsolver_weights"
  Data Type Conversion19/1 -> Bus Creator2/5  "Istunt_state"
  Bus Selector1/6 -> Mux/6  "<z>"
  Bus Selector6/1 -> Data Type Conversion4/1  "<data>"
  FF Input/2 -> Bus Selector1/1
  Bus Selector1/3 -> Mux/3  "<z>"
  Bus Selector2/2 -> Mux1/2  "<y>"
  Bus Selector2/8 -> Mux2/1  "<x>"
  Bus Selector1/5 -> Mux/5  "<y>"
  Bus Selector9/1 -> Data Type Conversion6/1  "<data>"
  Subscribe/2 -> Bus Selector/1
  Subscribe8/2 -> Bus Selector9/1
  Bus Selector10/1 -> Mux4/1  "<x>"
  Bus Selector2/10 -> Mux2/3  "<z>"
  Bus Selector10/2 -> Mux4/2  "<y>"
  Subscribe5/2 -> Bus Selector6/1
  Mux1/1 -> Current State/1  "DApose"
  Mux2/1 -> Current State/2  "DAtwist"
  Mux3/1 -> Desired Pose/2  "DAdesired_pose"
  Bus Selector3/1 -> Data Type Conversion2/1  "<mode>"
  Bus Selector5/5 -> Data Type Conversion1/1  "<mode>"
  Bus Creator2/1 -> Message Bus/1
  Current State/1 -> Bus Creator2/1  "current_state"
  Desired Pose/1 -> Bus Creator2/2  "desired_pose"
  Bus Selector4/1 -> Data Type Conversion3/1  "<data>"
  Bus Creator/1 -> Bus Creator2/4  "teleop"
  Bus Creator1/1 -> Bus Creator2/6  "thruster_solver"
  Data Type Conversion1/1 -> Desired Pose/3  "Iangular_mode"
  Data Type Conversion2/1 -> Desired Pose/1  "Ilinear_mode"
  Data Type Conversion3/1 -> Bus Creator2/3  "Bmotion_enabled"
  Data Type Conversion4/1 -> Bus Creator/1  "Dthrottle"
  Data Type Conversion5/1 -> Bus Creator/2  "Dreverse_throttle"
  Data Type Conversion6/1 -> Bus Creator/3  "Btrigger_boost"
  Data Type Conversion7/1 -> Bus Creator/4  "Djoy_R_X"
  Mux5/1 -> Current State/3  "DAtwist_accel"
  Subscribe11/2 -> Bus Selector12/1
  Bus Selector12/1 -> Mux5/1  "<x>"
  Bus Selector12/6 -> Mux5/6  "<z>"
  Bus Selector12/5 -> Mux5/5  "<y>"
  Bus Selector12/4 -> Mux5/4  "<x>"
  Bus Selector12/3 -> Mux5/3  "<y>"
  Bus Selector12/2 -> Mux5/2  "<z>"
  Subscribe12/1 -> Bus Creator2/7  "re_init"
  Bus Selector2/6 -> Mux1/6  "<z>"
  Bus Selector2/3 -> Mux1/3  "<z>"

== matlab function trial/Subsystem/MATLAB Function ==
  data: currentPositions input; world2Body output
function world2Body = fcn(currentPositions)
quat = [currentPositions(7), currentPositions(4),currentPositions(5), currentPositions(6)];

world2Body = transpose(quat2rotm(quat));
